simulink subsystem "State_Machine_MM"  (R2023b)
settings: Solver=VariableStepAuto  StartTime=0.0  StopTime=10.0  RelTol=1e-3
undefined symbols (not defined in the file): lb_mm, nF, ub_mm
libraries: dspstat3 x1
settings Model: Creator=Inver  LastModifiedBy=Inver

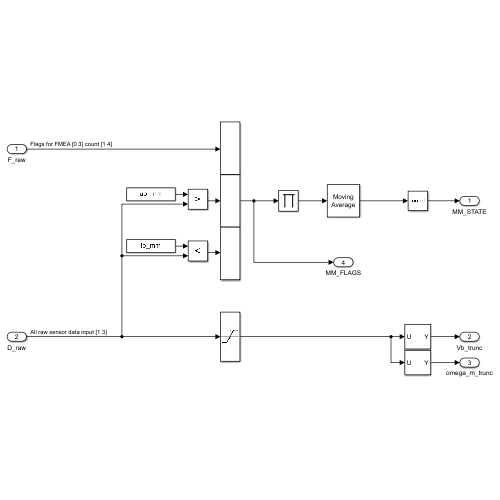
[thumbnail: Simulink's stored preview of the top-level diagram]
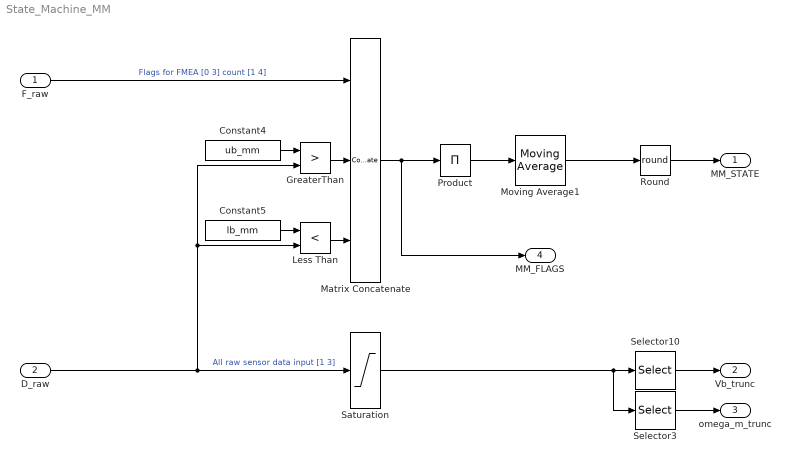
== system State_Machine_MM ==
  F_raw : Inport
  D_raw : Inport  Port=2
  Constant4 : Constant  Value=ub_mm
  Constant5 : Constant  Value=lb_mm
  GreaterThan : RelationalOperator  Operator=>  OutDataTypeStr=boolean  RndMeth=Simplest  InputSameDT=off
  Less Than : RelationalOperator  Operator=<  OutDataTypeStr=boolean  RndMeth=Simplest  InputSameDT=off
  Matrix Concatenate : Concatenate  NumInputs=3  ConcatenateDimension=2
  Moving Average1 : dspstat3/Moving Average  Method=Sliding window  ForgettingFactorPort=off  SpecifyWindowLength=on  WindowLength=nF  OverlapLength=nF-1  AllowArbitraryInputLength=off  ForgettingFactor=0.9  SimulateUsing=Code generation
  Product : Product  Inputs=1  OutDataTypeStr=double  SaturateOnIntegerOverflow=on
  Round : Rounding  Operator=round
  Saturation : Saturate  UpperLimit=ub_mm  LowerLimit=lb_mm
  Selector10 : Selector  IndexMode=Zero-based  InputPortWidth=19  IndexOptions=Index vector (dialog)  Indices=0  OutputSizes=1
  Selector3 : Selector  IndexMode=Zero-based  InputPortWidth=19  IndexOptions=Index vector (dialog)  Indices=[1 2]  OutputSizes=1
  MM_STATE : Outport
  Vb_trunc : Outport  Port=2
  omega_m_trunc : Outport  Port=3
  MM_FLAGS : Outport  Port=4
  wires:
  Matrix Concatenate/1 -> MM_FLAGS/1, Product/1
  Round/1 -> MM_STATE/1
  Selector10/1 -> Vb_trunc/1
  Selector3/1 -> omega_m_trunc/1
  Saturation/1 -> Selector10/1, Selector3/1
  Moving Average1/1 -> Round/1
  Product/1 -> Moving Average1/1
  D_raw/1 -> Less Than/2, GreaterThan/2, Saturation/1  "All raw sensor data input [1 3]"
  Constant5/1 -> Less Than/1
  Constant4/1 -> GreaterThan/1
  GreaterThan/1 -> Matrix Concatenate/2
  Less Than/1 -> Matrix Concatenate/3
  F_raw/1 -> Matrix Concatenate/1  "Flags for FMEA [0 3] count [1 4]"
